simulink model "testing_platform_continuous_reaction_linearization"  (Simulink 7.9)
settings: Solver=ode45  StartTime=0.0  StopTime=10.0  RelTol=1e-3
values from neighbouring files (symbols this model uses):
  coeff = block.DialogPrm(1).Data    [continuous_reaction_model.m]    (also in continuous_reaction_model_scaled.m; continuous_reaction_model_scaled_sensitivity.m)
  x0 = block.DialogPrm(2).Data    [continuous_reaction_model.m]    (also in continuous_reaction_model_scaled.m; continuous_reaction_model_scaled_sensitivity.m)
settings Model: Creator=marco  LastModifiedBy=marco

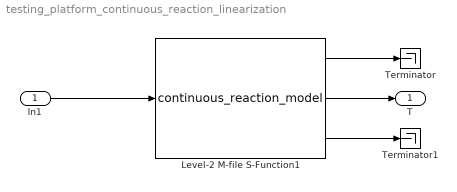
== system testing_platform_continuous_reaction_linearization ==
  In1 : Inport
  Level-2 M-file S-Function1 : M-S-Function  FunctionName=continuous_reaction_model  Parameters=coeff x0
  Terminator : Terminator
  Terminator1 : Terminator
  T : Outport
  wires:
  In1/1 -> Level-2 M-file S-Function1/1
  Level-2 M-file S-Function1/2 -> T/1
  Level-2 M-file S-Function1/1 -> Terminator/1
  Level-2 M-file S-Function1/3 -> Terminator1/1
